simulink model "nonlinear"
settings: Solver=ode45  StartTime=0.0  StopTime=10.0  RelTol=1e-3
values from neighbouring files (symbols this model uses):
  b = ku/k    [glabatom.m]    (also in matlab.mat = 0.251206720988)
  delta = Jp*zeta*omegan    [glabatom.m]    (also in matlab.mat = 0.000181694248674)
  Jp = m*g*l/(omegan^2)    [glabatom.m]    (also in matlab.mat = 0.00388561360108)
  k1 = T*b    [main.m]    (also in matlab.mat = 0.0401930753581; stavova_zpetna.m)
  k2 = eval(k2)    [main.m]    (also in matlab.mat = 0.00595; stavova_zpetna.m)
  k3 = eval(k3)    [main.m]    (also in matlab.mat = 0.2918475; stavova_zpetna.m)
settings Model: Creator=student  LastModifiedBy=matous
settings DataIOCC: LimitDataPoints=on  SaveFormat=Array  ReturnWorkspaceOutputs=off
settings OptimizationCC: LifeSpan=inf  SimCompilerOptimization=Off
settings DebuggingCC: SolverPrmCheckMsg=warning  MultiTaskDSMMsg=warning  MultiTaskCondExecSysMsg=none  FcnCallInpInsideContextMsg=Enable All  FrameProcessingCompatibilityMsg=warning  StrictBusMsg=None  SFUnexpectedBacktrackingDiag=warning  SFNoUnconditionalDefaultTransitionDiag=warning
settings HardwareCC: ProdBitPerPointer=32  ProdLargestAtomicFloat=None  ProdIntDivRoundTo=Undefined  ProdEndianess=Unspecified  ProdWordSize=32  ProdHWDeviceType=32-bit Generic
settings ModelReferenceCC: PropagateSignalLabelsOutOfModel=off
settings SFSimCC: SimUseLocalCustomCode=off
settings RTWCC: RTWUseLocalCustomCode=off  IncludeERTFirstTime=on  RTWCompilerOptimization=Off
settings GRTTargetCC: GeneratePreprocessorConditionals=Disable all

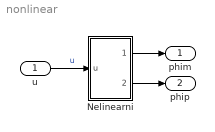
== system nonlinear ==
  u : Inport
  Nelinearni : Subsystem
  phim : Outport
  phip : Outport  Port=2
  wires:
  u/1 -> Nelinearni/1(u)  "u"
  Nelinearni/1(phim) -> phim/1
  Nelinearni/2(phip) -> phip/1

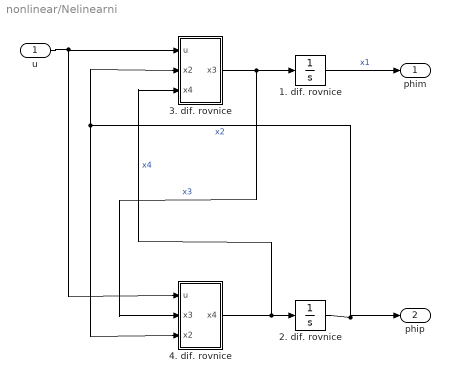
== system nonlinear/Nelinearni ==
  u : Inport
  1. dif. rovnice : Integrator
  2. dif. rovnice : Integrator
  3. dif. rovnice : Subsystem
  4. dif. rovnice : Subsystem
  phim : Outport
  phip : Outport  Port=2
  wires:
  1. dif. rovnice/1 -> phim/1  "x1"
  4. dif. rovnice/1(x4) -> 3. dif. rovnice/3(x4), 2. dif. rovnice/1  "x4"
  2. dif. rovnice/1 -> phip/1, 4. dif. rovnice/3(x2), 3. dif. rovnice/2(x2)  "x2"
  3. dif. rovnice/1(x3) -> 4. dif. rovnice/2("x3 "), 1. dif. rovnice/1  "x3"
  u/1 -> 4. dif. rovnice/1(u), 3. dif. rovnice/1(u)

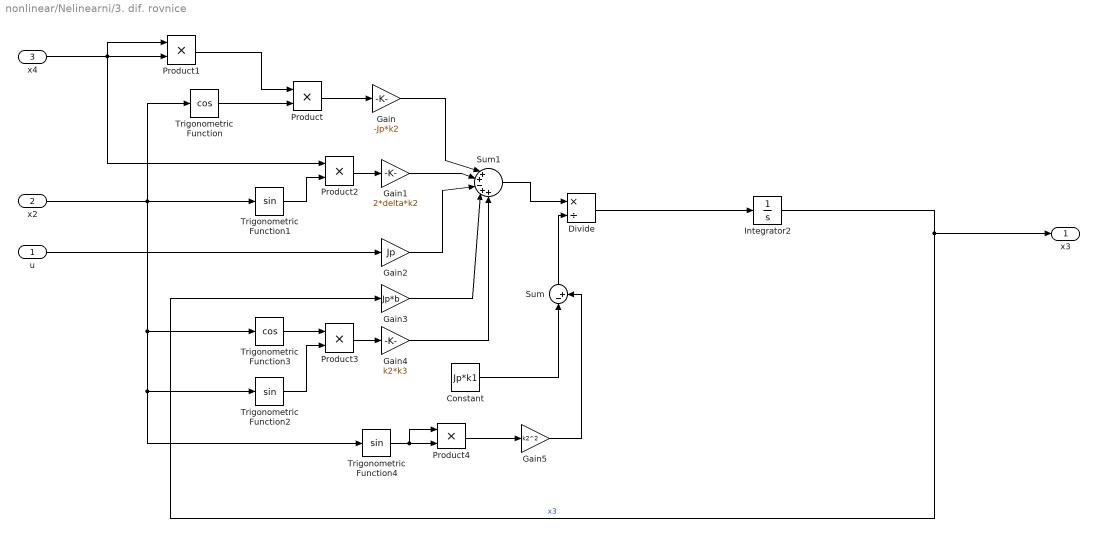
== system nonlinear/Nelinearni/3. dif. rovnice ==
  u : Inport
  x2 : Inport  Port=2
  x4 : Inport  Port=3
  Constant : Constant  Value=Jp*k1
  Divide : Product  Inputs=*/
  Gain : Gain  Gain=-Jp*k2
  Gain1 : Gain  Gain=2*delta*k2
  Gain2 : Gain  Gain=Jp
  Gain3 : Gain  Gain=Jp*b
  Gain4 : Gain  Gain=k2*k3
  Gain5 : Gain  Gain=k2^2
  Integrator2 : Integrator
  Product{,1..4} (5 alike) : Product
  Sum : Sum  Inputs=|-+
  Sum1 : Sum  Inputs=|++-++
  Trigonometric Function : Trigonometry  Operator=cos
  Trigonometric Function1 : Trigonometry
  Trigonometric Function2 : Trigonometry
  Trigonometric Function3 : Trigonometry  Operator=cos
  Trigonometric Function4 : Trigonometry
  x3 : Outport
  wires:
  Trigonometric Function3/1 -> Product3/1
  Divide/1 -> Integrator2/1
  x2/1 -> Trigonometric Function4/1, Trigonometric Function2/1, Trigonometric Function3/1, Trigonometric Function1/1, Trigonometric Function/1
  Product3/1 -> Gain4/1
  Trigonometric Function2/1 -> Product3/2
  Gain4/1 -> Sum1/5
  Gain/1 -> Sum1/1
  Product2/1 -> Gain1/1
  Trigonometric Function1/1 -> Product2/2
  u/1 -> Gain2/1
  Gain3/1 -> Sum1/4
  Gain1/1 -> Sum1/2
  Gain2/1 -> Sum1/3
  Sum1/1 -> Divide/1
  Product/1 -> Gain/1
  Sum/1 -> Divide/2
  x4/1 -> Product1/2, Product2/1, Product1/1
  Product1/1 -> Product/1
  Integrator2/1 -> Gain3/1, x3/1  "x3"
  Trigonometric Function/1 -> Product/2
  Gain5/1 -> Sum/2
  Constant/1 -> Sum/1
  Product4/1 -> Gain5/1
  Trigonometric Function4/1 -> Product4/1, Product4/2

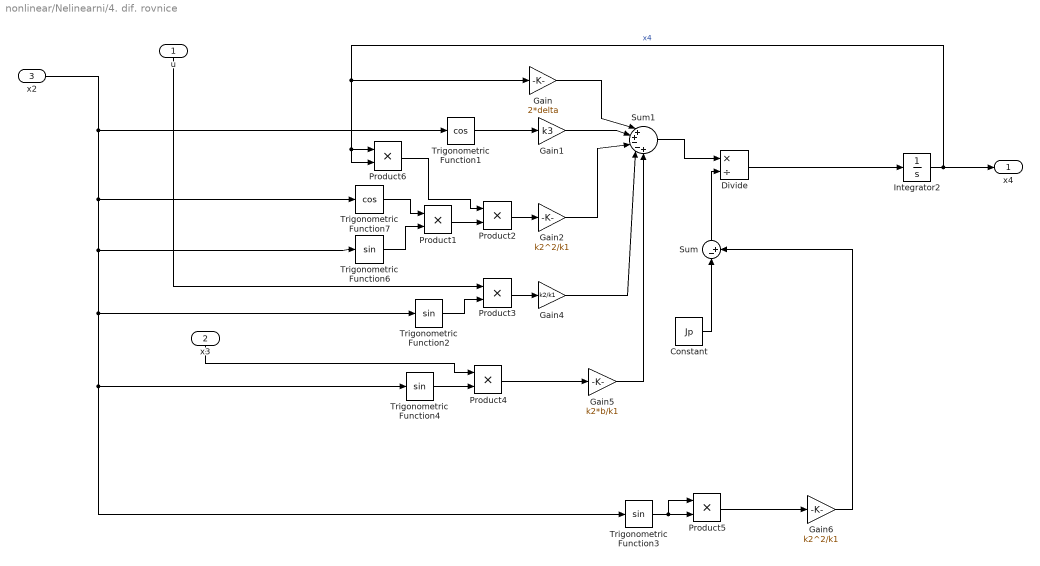
== system nonlinear/Nelinearni/4. dif. rovnice ==
  u : Inport
  "x3 " : Inport  Port=2
  x2 : Inport  Port=3
  Constant : Constant  Value=Jp
  Divide : Product  Inputs=*/
  Gain : Gain  Gain=2*delta
  Gain1 : Gain  Gain=k3
  Gain2 : Gain  Gain=k2^2/k1
  Gain4 : Gain  Gain=k2/k1
  Gain5 : Gain  Gain=k2*b/k1
  Gain6 : Gain  Gain=k2^2/k1
  Integrator2 : Integrator
  Product{1..6} (6 alike) : Product
  Sum : Sum  Inputs=|-+
  Sum1 : Sum  Inputs=|++--+
  Trigonometric Function1 : Trigonometry  Operator=cos
  Trigonometric Function{2..4,6} (4 alike) : Trigonometry
  Trigonometric Function7 : Trigonometry  Operator=cos
  x4 : Outport
  wires:
  Trigonometric Function3/1 -> Product5/1, Product5/2
  Product5/1 -> Gain6/1
  Divide/1 -> Integrator2/1
  Product3/1 -> Gain4/1
  Gain/1 -> Sum1/1
  Constant/1 -> Sum/1
  Gain6/1 -> Sum/2
  Integrator2/1 -> x4/1, Gain/1, Product6/1, Product6/2  "x4"
  Sum/1 -> Divide/2
  Product4/1 -> Gain5/1
  Sum1/1 -> Divide/1
  Gain2/1 -> Sum1/3
  Gain1/1 -> Sum1/2
  Trigonometric Function1/1 -> Gain1/1
  Trigonometric Function2/1 -> Product3/2
  Trigonometric Function6/1 -> Product1/2
  Trigonometric Function7/1 -> Product1/1
  Gain5/1 -> Sum1/5
  Trigonometric Function4/1 -> Product4/2
  Gain4/1 -> Sum1/4
  Product2/1 -> Gain2/1
  u/1 -> Product3/1
  x2/1 -> Trigonometric Function1/1, Trigonometric Function7/1, Trigonometric Function6/1, Trigonometric Function3/1, Trigonometric Function4/1, Trigonometric Function2/1
  "x3 "/1 -> Product4/1
  Product1/1 -> Product2/2
  Product6/1 -> Product2/1
